simulink model "diffrelay"  (Simulink 8.5)
settings: Solver=ode45  SolverMode=SingleTasking  StartTime=0.0  StopTime=1.0  RelTol=1e-3  AbsTol=1e-6
undefined symbols (not defined in the file or in its folder): Time
libraries: elements x51
settings Model: Creator=PC  LastModifiedBy=PC  ExtModeTrigMode=oneshot  ExtModeArmWhenConnect=off
settings DataIOCC: LimitDataPoints=off
settings OptimizationCC: BlockReduction=off  BooleanDataType=off  ExpressionDepthLimit=128
settings DebuggingCC: SaveWithParameterizedLinksMsg=none  SignalResolutionControl=TryResolveAllWithWarning  MultiTaskDSMMsg=warning  MultiTaskCondExecSysMsg=none  FcnCallInpInsideContextMsg=EnableAllAsError  StateNameClashWarn=none
settings HardwareCC: TargetUnknown=on

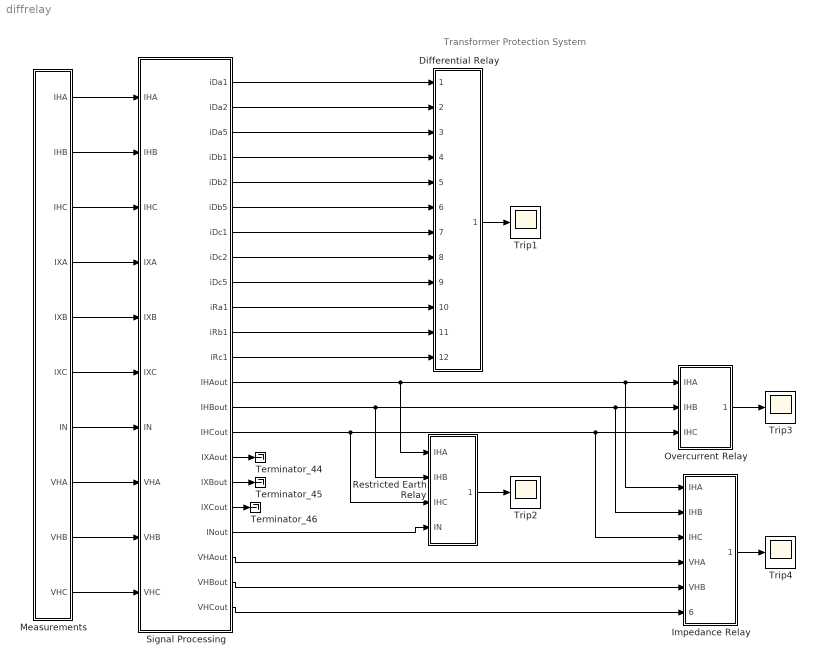
== system diffrelay ==
  note: Transformer Protection System
  Differential Relay : Subsystem  mask(Differential Relay){y2=300, x2=1000, y1=100, x1=500, c5=0.15, c2=0.15, unbiased=1e6, pickup=1}
      mask prompts: y2 "Biased Characteristic Point: D2"; x2 "Biased Characteristic Point: R2"; y1 "Biased Characteristic Point: D1"; x1 "Biased Characteristic Point: R1"; c5 "Fifth Harmonics Restraint Parameter"; c2 "Second Harmonics Restraint Parameter"; unbiased "Unbiased Threshold Value"; pickup "Pickup Value"
      mask help: Two-slope bias characteristic, instantaneous unbiased differential overcurrent element, second and fifth harmonic restraints.
  Impedance Relay : Subsystem  mask(Six-element Three-zone Impedance Relay){r=[0 0; -60 0; -65 -65; 0 -60], z2=[0 -0.5 ;1 0; 2 40; -0.5 0], z1=[0 -0.5 ;0.6 0; 1 21; -0.5 0]}
      mask prompts: r "Backward Zone Setting"; z2 "Zone 2 Setting"; z1 "Zone 1 Setting"
      mask help: Six-element three-zone (two forward and one backward) impedance relays for the backup protection of the high voltage winding.
  Measurements : Subsystem
  Overcurrent Relay : Subsystem  mask(Three-phase Inverse-time Overcurrent Relay){k=0.02, reset=0.9, pickupv=500}
      mask prompts: k "Time Parameter"; reset "Ratio of Reset to pick up"; pickupv "Pick-up Value"
      mask help: Three-phase inverse-time overcurrent relays for the back-up protection of the high voltage winding.
  Restricted Earth Relay : Subsystem  mask(Restricted Earth Protection for the Wye-connected Winding){rc=1, pickup0=0.5, zot=2100, k=0.2, choice=Differential}
      mask prompts: rc "Ratio Mismatch Compensation"; pickup0 "Zero Differential Pick-up Value"; zot "Zero Sequence Overcurrent Threshold"; k "Biased Parameter"; choice "Type of protection"
      mask help: Zero sequence overcurrent protection and zero sequence differential protection.
      mask TypeOptions choice: Overcurrent | Differential
  Signal Processing : Subsystem  mask(Signal Processing){ctx=31.5, cth=1.38, vs=13.8e3, vp=315e3, vector=11}
      mask prompts: ctx "CT Ratio of Low Voltage Side"; cth "CT Ratio of High Voltage Side"; vs "Secondary Voltage"; vp "Primary Voltage"; vector "Transformer Connection Vector"
      mask help: Transform analog measurements to digital format, including filtering, sampling . . .
  Terminator_44 : Terminator
  Terminator_45 : Terminator
  Terminator_46 : Terminator
  Trip{1..4} (4 alike) : Scope
      Trip1 settings: YMin=-1  YMax=1
      Trip2 settings: YMin=-2  YMax=2
      Trip3 settings: YMin=-1  YMax=1
      Trip4 settings: YMin=-1  YMax=1
  wires:
  Measurements/1(IHA) -> Signal Processing/1(IHA)
  Signal Processing/1(iDa1) -> Differential Relay/1(IDa1)
  Signal Processing/2(iDa2) -> Differential Relay/2(IDa2)
  Signal Processing/7(iDc1) -> Differential Relay/7(IDc1)
  Signal Processing/8(iDc2) -> Differential Relay/8(IDc2)
  Signal Processing/12(iRc1) -> Differential Relay/12(IRc1)
  Signal Processing/11(iRb1) -> Differential Relay/11(IRb1)
  Signal Processing/10(iRa1) -> Differential Relay/10(IRa1)
  Signal Processing/9(iDc5) -> Differential Relay/9(IDc5)
  Signal Processing/16(IXAout) -> Terminator_44/1
  Signal Processing/17(IXBout) -> Terminator_45/1
  Signal Processing/18(IXCout) -> Terminator_46/1
  Signal Processing/19(INout) -> Restricted Earth Relay/4(IN)
  Signal Processing/13(IHAout) -> Restricted Earth Relay/1(IHA), Overcurrent Relay/1(IHA), Impedance Relay/1(IHA)
  Signal Processing/14(IHBout) -> Restricted Earth Relay/2(IHB), Overcurrent Relay/2(IHB), Impedance Relay/2(IHB)
  Signal Processing/15(IHCout) -> Restricted Earth Relay/3(IHC), Overcurrent Relay/3(IHC), Impedance Relay/3(IHC)
  Signal Processing/20(VHAout) -> Impedance Relay/4(VHA)
  Signal Processing/21(VHBout) -> Impedance Relay/5(VHB)
  Signal Processing/22(VHCout) -> Impedance Relay/6(VHC)
  Measurements/2(IHB) -> Signal Processing/2(IHB)
  Measurements/3(IHC) -> Signal Processing/3(IHC)
  Measurements/4(IXA) -> Signal Processing/4(IXA)
  Measurements/5(IXB) -> Signal Processing/5(IXB)
  Measurements/6(IXC) -> Signal Processing/6(IXC)
  Measurements/7(IN) -> Signal Processing/7(IN)
  Measurements/8(VHA) -> Signal Processing/8(VHA)
  Measurements/9(VHB) -> Signal Processing/9(VHB)
  Measurements/10(VHC) -> Signal Processing/10(VHC)
  Differential Relay/1(Trip1) -> Trip1/1
  Overcurrent Relay/1(Trip 3) -> Trip3/1
  Restricted Earth Relay/1(Trip 2) -> Trip2/1
  Impedance Relay/1(Trip4) -> Trip4/1
  Signal Processing/3(iDa5) -> Differential Relay/3(IDa5)
  Signal Processing/4(iDb1) -> Differential Relay/4(IDb1)
  Signal Processing/5(iDb2) -> Differential Relay/5(IDb2)
  Signal Processing/6(iDb5) -> Differential Relay/6(IDb5)

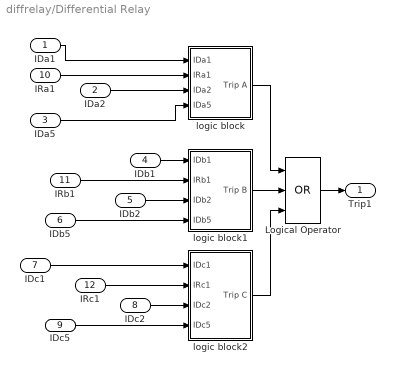
== system diffrelay/Differential Relay ==
  IDa1 : Inport
  IDa2 : Inport  Port=2
  IDa5 : Inport  Port=3
  IDb1 : Inport  Port=4
  IDb2 : Inport  Port=5
  IDb5 : Inport  Port=6
  IDc1 : Inport  Port=7
  IDc2 : Inport  Port=8
  IDc5 : Inport  Port=9
  IRa1 : Inport  Port=10
  IRb1 : Inport  Port=11
  IRc1 : Inport  Port=12
  Logical Operator : Logic  Operator=OR  Inputs=3
  logic block : Subsystem
  logic block1 : Subsystem
  logic block2 : Subsystem
  Trip1 : Outport
  wires:
  logic block/1(Trip A) -> Logical Operator/1
  logic block1/1(Trip B) -> Logical Operator/2
  logic block2/1(Trip C) -> Logical Operator/3
  Logical Operator/1 -> Trip1/1
  IRc1/1 -> logic block2/2(IRc1)
  IRb1/1 -> logic block1/2(IRb1)
  IDc5/1 -> logic block2/4(IDc5)
  IDc2/1 -> logic block2/3(IDc2)
  IDb2/1 -> logic block1/3(IDb2)
  IDb1/1 -> logic block1/1(IDb1)
  IDa5/1 -> logic block/4(IDa5)
  IDa2/1 -> logic block/3(IDa2)
  IDa1/1 -> logic block/1(IDa1)
  IRa1/1 -> logic block/2(IRa1)
  IDc1/1 -> logic block2/1(IDc1)
  IDb5/1 -> logic block1/4(IDb5)

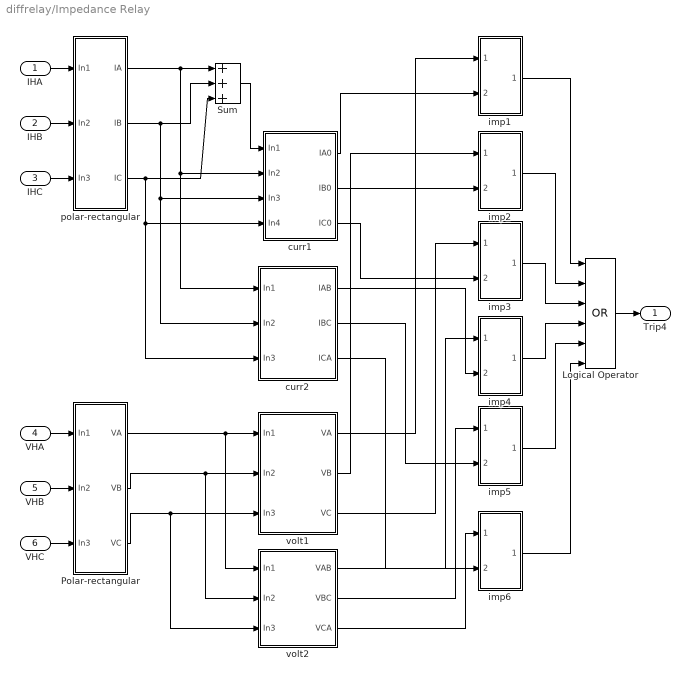
== system diffrelay/Impedance Relay ==
  IHA : Inport
  IHB : Inport  Port=2
  IHC : Inport  Port=3
  VHA : Inport  Port=4
  VHB : Inport  Port=5
  VHC : Inport  Port=6
  " curr1" : Subsystem
  Logical Operator : Logic  Operator=OR  Inputs=6
  Polar-rectangular : Subsystem
  Sum : Sum  Inputs=+++  SaturateOnIntegerOverflow=on  InputSameDT=on  OutDataTypeStr=Inherit: Same as first input
  curr2 : Subsystem
  imp1 : Subsystem
  imp2 : Subsystem
  imp3 : Subsystem
  imp4 : Subsystem
  imp5 : Subsystem
  imp6 : Subsystem
  polar-rectangular : Subsystem
  volt1 : Subsystem
  volt2 : Subsystem
  Trip4 : Outport
  wires:
  " curr1"/1(IA0) -> imp1/2(In2)
  polar-rectangular/1(IA) -> Sum/1, " curr1"/2(In2), curr2/1(In1)
  volt1/1(VA) -> imp1/1(In1)
  Polar-rectangular/1(VA) -> volt1/1(In1), volt2/1(In1)
  Polar-rectangular/2(VB) -> volt1/2(In2), volt2/2(In2)
  polar-rectangular/2(IB) -> Sum/2, " curr1"/3(In3), curr2/2(In2)
  polar-rectangular/3(IC) -> Sum/3, " curr1"/4(In4), curr2/3(In3)
  Polar-rectangular/3(VC) -> volt1/3(In3), volt2/3(In3)
  Sum/1 -> " curr1"/1(In1)
  imp1/1(e1trip) -> Logical Operator/1
  imp2/1(e2trip) -> Logical Operator/2
  imp3/1(e3trip) -> Logical Operator/3
  imp4/1(e4trip) -> Logical Operator/4
  imp5/1(e5trip) -> Logical Operator/5
  imp6/1(e6trip) -> Logical Operator/6
  Logical Operator/1 -> Trip4/1
  " curr1"/2(IB0) -> imp2/2(In2)
  volt1/2(VB) -> imp2/1(In1)
  volt1/3(VC) -> imp3/1(In1)
  " curr1"/3(IC0) -> imp3/2(In2)
  volt2/1(VAB) -> imp4/1(In1)
  curr2/1(IAB) -> imp4/2(In2)
  volt2/2(VBC) -> imp5/1(In1)
  curr2/2(IBC) -> imp5/2(In2)
  volt2/3(VCA) -> imp6/1(In1)
  curr2/3(ICA) -> imp6/2(In2)
  IHA/1 -> polar-rectangular/1(In1)
  IHB/1 -> polar-rectangular/2(In2)
  IHC/1 -> polar-rectangular/3(In3)
  VHA/1 -> Polar-rectangular/1(In1)
  VHB/1 -> Polar-rectangular/2(In2)
  VHC/1 -> Polar-rectangular/3(In3)

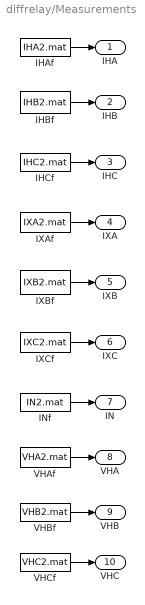
== system diffrelay/Measurements ==
  IHAf : FromFile  FileName=IHA2.mat  SampleTime=0
  IHBf : FromFile  FileName=IHB2.mat  SampleTime=0
  IHCf : FromFile  FileName=IHC2.mat  SampleTime=0
  INf : FromFile  FileName=IN2.mat  SampleTime=0
  IXAf : FromFile  FileName=IXA2.mat  SampleTime=0
  IXBf : FromFile  FileName=IXB2.mat  SampleTime=0
  IXCf : FromFile  FileName=IXC2.mat  SampleTime=0
  VHAf : FromFile  FileName=VHA2.mat  SampleTime=0
  VHBf : FromFile  FileName=VHB2.mat  SampleTime=0
  VHCf : FromFile  FileName=VHC2.mat  SampleTime=0
  IHA : Outport
  IHB : Outport  Port=2
  IHC : Outport  Port=3
  IXA : Outport  Port=4
  IXB : Outport  Port=5
  IXC : Outport  Port=6
  IN : Outport  Port=7
  VHA : Outport  Port=8
  VHB : Outport  Port=9
  VHC : Outport  Port=10
  wires:
  IHAf/1 -> IHA/1
  IHBf/1 -> IHB/1
  IHCf/1 -> IHC/1
  IXAf/1 -> IXA/1
  IXBf/1 -> IXB/1
  IXCf/1 -> IXC/1
  INf/1 -> IN/1
  VHAf/1 -> VHA/1
  VHBf/1 -> VHB/1
  VHCf/1 -> VHC/1

== system diffrelay/Overcurrent Relay ==
  IHA : Inport
  IHB : Inport  Port=2
  IHC : Inport  Port=3
  Demux : Demux  Outputs=2
  Demux1 : Demux  Outputs=2
  Demux2 : Demux  Outputs=2
  Logical Operator : Logic  Operator=OR  Inputs=3
  UCA : elements/UC  type0=Signal-Time  sign=>  Ipickup=pickupv  k1=reset  type1=Very Inverse  type3=integration  k=k  fs=32*60
  UCB : elements/UC  type0=Signal-Time  sign=>  Ipickup=pickupv  k1=reset  type1=Very Inverse  type3=integration  k=k  fs=32*60
  UCC : elements/UC  type0=Signal-Time  sign=>  Ipickup=pickupv  k1=reset  type1=Very Inverse  type3=integration  k=k  fs=32*60
  Trip 3 : Outport
  wires:
  Demux2/1 -> UCC/1
  Demux1/1 -> UCB/1
  Demux/1 -> UCA/1
  UCA/1 -> Logical Operator/1
  UCB/1 -> Logical Operator/2
  UCC/1 -> Logical Operator/3
  Logical Operator/1 -> Trip 3/1
  IHA/1 -> Demux/1
  IHB/1 -> Demux1/1
  IHC/1 -> Demux2/1
  Demux/2 -> UCA/2
  Demux1/2 -> UCB/2
  Demux2/2 -> UCC/2

== system diffrelay/Restricted Earth Relay ==
  IHA : Inport
  IHB : Inport  Port=2
  IHC : Inport  Port=3
  IN : Inport  Port=4
  Choice : Constant  Value=choice
  Switch : Switch  Threshold=1.5  SaturateOnIntegerOverflow=on  InputSameDT=on
  Zero Sequence Differential : Subsystem
  Zero Sequence  Overcurrent : Subsystem
  rc : Gain  Gain=rc  SaturateOnIntegerOverflow=on  OutDataTypeStr=Inherit: Same as input  ParamDataTypeStr=Inherit: Same as input
  Trip 2 : Outport
  wires:
  Choice/1 -> Switch/2
  Zero Sequence Differential/1(Out1) -> Switch/1
  Switch/1 -> Trip 2/1
  Zero Sequence  Overcurrent/1(Out1) -> Switch/3
  IHA/1 -> Zero Sequence Differential/1(IHA)
  IHB/1 -> Zero Sequence Differential/2(IHB)
  IHC/1 -> Zero Sequence Differential/3(IHC)
  IN/1 -> Zero Sequence  Overcurrent/1(In1), rc/1
  rc/1 -> Zero Sequence Differential/4(IN)

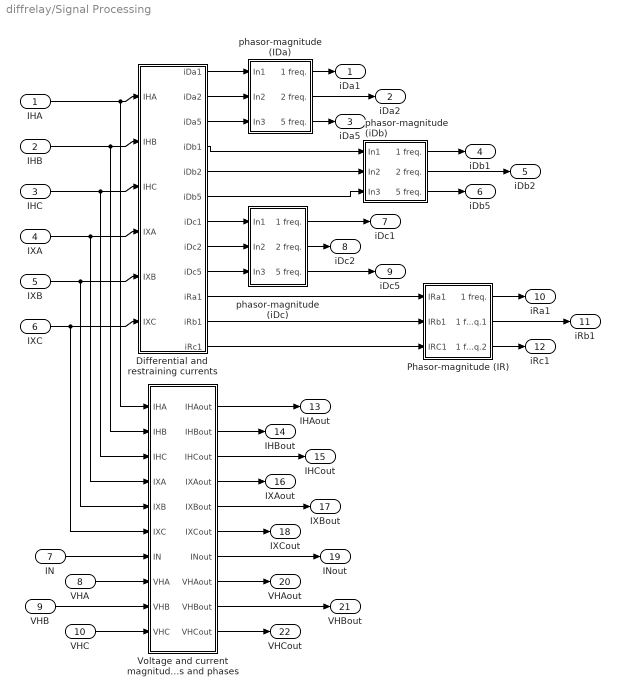
== system diffrelay/Signal Processing ==
  IHA : Inport
  IHB : Inport  Port=2
  IHC : Inport  Port=3
  IXA : Inport  Port=4
  IXB : Inport  Port=5
  IXC : Inport  Port=6
  IN : Inport  Port=7
  VHA : Inport  Port=8
  VHB : Inport  Port=9
  VHC : Inport  Port=10
  Differential and  restraining currents : Subsystem
  Phasor-magnitude (IR) : Subsystem
  Voltage and current magnitudes and phases : Subsystem
  phasor-magnitude (IDa) : Subsystem
  phasor-magnitude (iDb) : Subsystem
  phasor-magnitude (iDc) : Subsystem
  iDa1 : Outport
  iDa2 : Outport  Port=2
  iDa5 : Outport  Port=3
  iDb1 : Outport  Port=4
  iDb2 : Outport  Port=5
  iDb5 : Outport  Port=6
  iDc1 : Outport  Port=7
  iDc2 : Outport  Port=8
  iDc5 : Outport  Port=9
  iRa1 : Outport  Port=10
  iRb1 : Outport  Port=11
  iRc1 : Outport  Port=12
  IHAout : Outport  Port=13
  IHBout : Outport  Port=14
  IHCout : Outport  Port=15
  IXAout : Outport  Port=16
  IXBout : Outport  Port=17
  IXCout : Outport  Port=18
  INout : Outport  Port=19
  VHAout : Outport  Port=20
  VHBout : Outport  Port=21
  VHCout : Outport  Port=22
  wires:
  IHA/1 -> Differential and  restraining currents/1(IHA), Voltage and current magnitudes and phases/1(IHA)
  IHB/1 -> Differential and  restraining currents/2(IHB), Voltage and current magnitudes and phases/2(IHB)
  IHC/1 -> Differential and  restraining currents/3(IHC), Voltage and current magnitudes and phases/3(IHC)
  IXA/1 -> Differential and  restraining currents/4(IXA), Voltage and current magnitudes and phases/4(IXA)
  IXB/1 -> Differential and  restraining currents/5(IXB), Voltage and current magnitudes and phases/5(IXB)
  IXC/1 -> Differential and  restraining currents/6(IXC), Voltage and current magnitudes and phases/6(IXC)
  Differential and  restraining currents/1(iDa1) -> phasor-magnitude (IDa)/1(In1)
  Differential and  restraining currents/2(iDa2) -> phasor-magnitude (IDa)/2(In2)
  Differential and  restraining currents/3(iDa5) -> phasor-magnitude (IDa)/3(In3)
  phasor-magnitude (IDa)/1(1 freq.) -> iDa1/1
  phasor-magnitude (IDa)/2(2 freq.) -> iDa2/1
  phasor-magnitude (IDa)/3(5 freq.) -> iDa5/1
  Differential and  restraining currents/4(iDb1) -> phasor-magnitude (iDb)/1(In1)
  Differential and  restraining currents/5(iDb2) -> phasor-magnitude (iDb)/2(In2)
  Differential and  restraining currents/6(iDb5) -> phasor-magnitude (iDb)/3(In3)
  phasor-magnitude (iDb)/1(1 freq.) -> iDb1/1
  phasor-magnitude (iDb)/2(2 freq.) -> iDb2/1
  phasor-magnitude (iDb)/3(5 freq.) -> iDb5/1
  Differential and  restraining currents/7(iDc1) -> phasor-magnitude (iDc)/1(In1)
  Differential and  restraining currents/8(iDc2) -> phasor-magnitude (iDc)/2(In2)
  Differential and  restraining currents/9(iDc5) -> phasor-magnitude (iDc)/3(In3)
  phasor-magnitude (iDc)/1(1 freq.) -> iDc1/1
  phasor-magnitude (iDc)/2(2 freq.) -> iDc2/1
  phasor-magnitude (iDc)/3(5 freq.) -> iDc5/1
  Differential and  restraining currents/10(iRa1) -> Phasor-magnitude (IR)/1(IRa1)
  Differential and  restraining currents/11(iRb1) -> Phasor-magnitude (IR)/2(IRb1)
  Differential and  restraining currents/12(iRc1) -> Phasor-magnitude (IR)/3(IRC1)
  Phasor-magnitude (IR)/1(1 freq.) -> iRa1/1
  Phasor-magnitude (IR)/2(1 freq.1) -> iRb1/1
  Phasor-magnitude (IR)/3(1 freq.2) -> iRc1/1
  Voltage and current magnitudes and phases/1(IHAout) -> IHAout/1
  Voltage and current magnitudes and phases/2(IHBout) -> IHBout/1
  Voltage and current magnitudes and phases/3(IHCout) -> IHCout/1
  Voltage and current magnitudes and phases/4(IXAout) -> IXAout/1
  Voltage and current magnitudes and phases/5(IXBout) -> IXBout/1
  Voltage and current magnitudes and phases/6(IXCout) -> IXCout/1
  Voltage and current magnitudes and phases/7(INout) -> INout/1
  Voltage and current magnitudes and phases/8(VHAout) -> VHAout/1
  Voltage and current magnitudes and phases/9(VHBout) -> VHBout/1
  Voltage and current magnitudes and phases/10(VHCout) -> VHCout/1
  IN/1 -> Voltage and current magnitudes and phases/7(IN)
  VHA/1 -> Voltage and current magnitudes and phases/8(VHA)
  VHB/1 -> Voltage and current magnitudes and phases/9(VHB)
  VHC/1 -> Voltage and current magnitudes and phases/10(VHC)

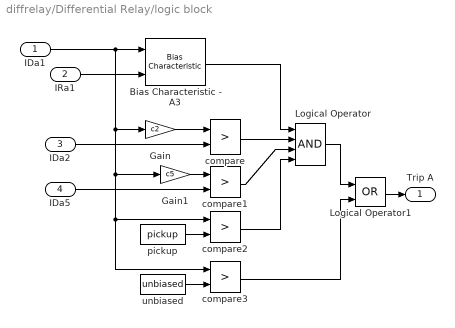
== system diffrelay/Differential Relay/logic block ==
  IDa1 : Inport
  IRa1 : Inport  Port=2
  IDa2 : Inport  Port=3
  IDa5 : Inport  Port=4
  Bias Characteristic - A3 : elements/Bias Characteristic  BC=[ 0 0; x1 y1; x2 y2 ]  fs=60*32
  Gain : Gain  Gain=c2  SaturateOnIntegerOverflow=on  OutDataTypeStr=Inherit: Same as input  ParamDataTypeStr=Inherit: Same as input
  Gain1 : Gain  Gain=c5  SaturateOnIntegerOverflow=on  OutDataTypeStr=Inherit: Same as input  ParamDataTypeStr=Inherit: Same as input
  Logical Operator : Logic  Inputs=4
  Logical Operator1 : Logic  Operator=OR
  compare{,1..3} (4 alike) : RelationalOperator  Operator=>  InputSameDT=on
  pickup : Constant  Value=pickup
  unbiased : Constant  Value=unbiased
  Trip A : Outport
  wires:
  Gain/1 -> compare/1
  Gain1/1 -> compare1/1
  pickup/1 -> compare2/2
  unbiased/1 -> compare3/2
  IDa2/1 -> compare/2
  IDa5/1 -> compare1/2
  Logical Operator1/1 -> Trip A/1
  Logical Operator/1 -> Logical Operator1/1
  compare3/1 -> Logical Operator1/2
  Bias Characteristic - A3/1 -> Logical Operator/1
  compare/1 -> Logical Operator/2
  compare1/1 -> Logical Operator/3
  compare2/1 -> Logical Operator/4
  IRa1/1 -> Bias Characteristic - A3/2
  IDa1/1 -> Bias Characteristic - A3/1, Gain/1, Gain1/1, compare2/1, compare3/1

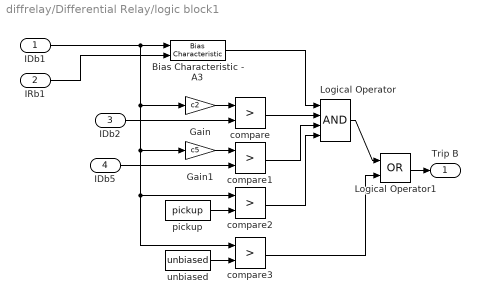
== system diffrelay/Differential Relay/logic block1 ==
  IDb1 : Inport
  IRb1 : Inport  Port=2
  IDb2 : Inport  Port=3
  IDb5 : Inport  Port=4
  Bias Characteristic - A3 : elements/Bias Characteristic  BC=[ 0 0; x1 y1; x2 y2 ]  fs=60*32
  Gain : Gain  Gain=c2  SaturateOnIntegerOverflow=on  OutDataTypeStr=Inherit: Same as input  ParamDataTypeStr=Inherit: Same as input
  Gain1 : Gain  Gain=c5  SaturateOnIntegerOverflow=on  OutDataTypeStr=Inherit: Same as input  ParamDataTypeStr=Inherit: Same as input
  Logical Operator : Logic  Inputs=4
  Logical Operator1 : Logic  Operator=OR
  compare{,1..3} (4 alike) : RelationalOperator  Operator=>  InputSameDT=on
  pickup : Constant  Value=pickup
  unbiased : Constant  Value=unbiased
  Trip B : Outport
  wires:
  IDb1/1 -> compare3/1, compare2/1, Gain1/1, Gain/1, Bias Characteristic - A3/1
  IRb1/1 -> Bias Characteristic - A3/2
  compare2/1 -> Logical Operator/4
  compare1/1 -> Logical Operator/3
  compare/1 -> Logical Operator/2
  Bias Characteristic - A3/1 -> Logical Operator/1
  compare3/1 -> Logical Operator1/2
  Logical Operator/1 -> Logical Operator1/1
  Logical Operator1/1 -> Trip B/1
  IDb5/1 -> compare1/2
  IDb2/1 -> compare/2
  unbiased/1 -> compare3/2
  pickup/1 -> compare2/2
  Gain1/1 -> compare1/1
  Gain/1 -> compare/1

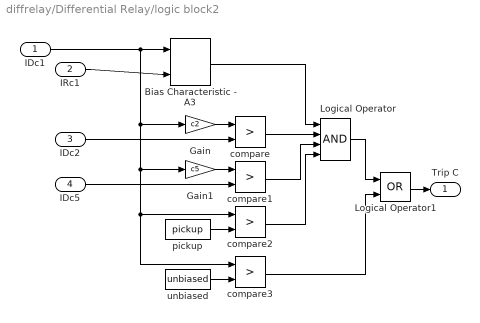
== system diffrelay/Differential Relay/logic block2 ==
  IDc1 : Inport
  IRc1 : Inport  Port=2
  IDc2 : Inport  Port=3
  IDc5 : Inport  Port=4
  Bias Characteristic - A3 : elements/Bias Characteristic  BC=[ 0 0; x1 y1; x2 y2 ]  fs=60*32
  Gain : Gain  Gain=c2  SaturateOnIntegerOverflow=on  OutDataTypeStr=Inherit: Same as input  ParamDataTypeStr=Inherit: Same as input
  Gain1 : Gain  Gain=c5  SaturateOnIntegerOverflow=on  OutDataTypeStr=Inherit: Same as input  ParamDataTypeStr=Inherit: Same as input
  Logical Operator : Logic  Inputs=4
  Logical Operator1 : Logic  Operator=OR
  compare{,1..3} (4 alike) : RelationalOperator  Operator=>  InputSameDT=on
  pickup : Constant  Value=pickup
  unbiased : Constant  Value=unbiased
  Trip C : Outport
  wires:
  Gain/1 -> compare/1
  Gain1/1 -> compare1/1
  pickup/1 -> compare2/2
  unbiased/1 -> compare3/2
  IDc2/1 -> compare/2
  IDc5/1 -> compare1/2
  Logical Operator1/1 -> Trip C/1
  Logical Operator/1 -> Logical Operator1/1
  compare3/1 -> Logical Operator1/2
  Bias Characteristic - A3/1 -> Logical Operator/1
  compare/1 -> Logical Operator/2
  compare1/1 -> Logical Operator/3
  compare2/1 -> Logical Operator/4
  IRc1/1 -> Bias Characteristic - A3/2
  IDc1/1 -> Bias Characteristic - A3/1, Gain/1, Gain1/1, compare2/1, compare3/1

== system diffrelay/Impedance Relay/ curr1 ==
  In1 : Inport
  In2 : Inport  Port=2
  In3 : Inport  Port=3
  In4 : Inport  Port=4
  C to M/A : Subsystem
  C to M/A1 : Subsystem
  C to M/A2 : Subsystem
  Sum1 : Sum  Inputs=2  SaturateOnIntegerOverflow=on  InputSameDT=on  OutDataTypeStr=Inherit: Same as first input
  Sum2 : Sum  Inputs=2  SaturateOnIntegerOverflow=on  InputSameDT=on  OutDataTypeStr=Inherit: Same as first input
  Sum3 : Sum  Inputs=2  SaturateOnIntegerOverflow=on  InputSameDT=on  OutDataTypeStr=Inherit: Same as first input
  IA0 : Outport
  IB0 : Outport  Port=2
  IC0 : Outport  Port=3
  wires:
  In1/1 -> Sum1/1, Sum2/1, Sum3/1
  Sum1/1 -> C to M/A/1(In1)
  In3/1 -> Sum2/2
  In2/1 -> Sum1/2
  Sum2/1 -> C to M/A1/1(In1)
  Sum3/1 -> C to M/A2/1(In1)
  In4/1 -> Sum3/2
  C to M/A/1(Out1) -> IA0/1
  C to M/A1/1(Out1) -> IB0/1
  C to M/A2/1(Out1) -> IC0/1

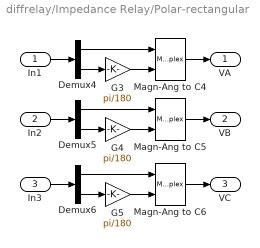
== system diffrelay/Impedance Relay/Polar-rectangular ==
  In1 : Inport
  In2 : Inport  Port=2
  In3 : Inport  Port=3
  Demux4 : Demux  Outputs=2
  Demux5 : Demux  Outputs=2
  Demux6 : Demux  Outputs=2
  G3 : Gain  Gain=pi/180  SaturateOnIntegerOverflow=on  OutDataTypeStr=Inherit: Same as input  ParamDataTypeStr=Inherit: Same as input
  G4 : Gain  Gain=pi/180  SaturateOnIntegerOverflow=on  OutDataTypeStr=Inherit: Same as input  ParamDataTypeStr=Inherit: Same as input
  G5 : Gain  Gain=pi/180  SaturateOnIntegerOverflow=on  OutDataTypeStr=Inherit: Same as input  ParamDataTypeStr=Inherit: Same as input
  Magn-Ang to C4 : MagnitudeAngleToComplex
  Magn-Ang to C5 : MagnitudeAngleToComplex
  Magn-Ang to C6 : MagnitudeAngleToComplex
  VA : Outport
  VB : Outport  Port=2
  VC : Outport  Port=3
  wires:
  Demux4/1 -> Magn-Ang to C4/1
  Demux4/2 -> G3/1
  G3/1 -> Magn-Ang to C4/2
  Demux5/2 -> G4/1
  G4/1 -> Magn-Ang to C5/2
  Demux5/1 -> Magn-Ang to C5/1
  Demux6/2 -> G5/1
  G5/1 -> Magn-Ang to C6/2
  Demux6/1 -> Magn-Ang to C6/1
  Magn-Ang to C4/1 -> VA/1
  In1/1 -> Demux4/1
  Magn-Ang to C5/1 -> VB/1
  In2/1 -> Demux5/1
  Magn-Ang to C6/1 -> VC/1
  In3/1 -> Demux6/1

== system diffrelay/Impedance Relay/curr2 ==
  In1 : Inport
  In2 : Inport  Port=2
  In3 : Inport  Port=3
  C to M/A : Subsystem
  C to M/A1 : Subsystem
  C to M/A2 : Subsystem
  Sum4 : Sum  Inputs=+-  SaturateOnIntegerOverflow=on  InputSameDT=on  OutDataTypeStr=Inherit: Same as first input
  Sum6 : Sum  Inputs=+-  SaturateOnIntegerOverflow=on  InputSameDT=on  OutDataTypeStr=Inherit: Same as first input
  Sum7 : Sum  Inputs=+-  SaturateOnIntegerOverflow=on  InputSameDT=on  OutDataTypeStr=Inherit: Same as first input
  IAB : Outport
  IBC : Outport  Port=2
  ICA : Outport  Port=3
  wires:
  In2/1 -> Sum4/2, Sum6/1
  In3/1 -> Sum6/2, Sum7/1
  In1/1 -> Sum4/1, Sum7/2
  Sum4/1 -> C to M/A/1(In1)
  C to M/A/1(Out1) -> IAB/1
  Sum6/1 -> C to M/A1/1(In1)
  C to M/A1/1(Out1) -> IBC/1
  Sum7/1 -> C to M/A2/1(In1)
  C to M/A2/1(Out1) -> ICA/1

== system diffrelay/Impedance Relay/imp1 ==
  In1 : Inport
  In2 : Inport  Port=2
   {,1,3..5} (5 alike) : Terminator
  BM : elements/BM  tpostv=none  plenv=4  tposti=none  pleni=4  tposts=none  plens=4  tpostz=none  plenz=4
  Logical Operator : Logic  Operator=OR  Inputs=3
  Time Delay1 : TransportDelay  DelayTime=0.2  BufferSize=2048
  Time Delay2 : TransportDelay  DelayTime=0.5  BufferSize=4096
  "ZC   " : elements/ZC     typez=Free expression  z1=z1  z2=z2  z3="[0  0; 0 0; 0 0; 0 0]"  z4="[0  0; 0 0; 0 0; 0 0]"  zr=r  fs=32*60
  e1trip : Outport
  wires:
  "ZC   "/2 -> Time Delay1/1
  "ZC   "/5 -> Time Delay2/1
  "ZC   "/3 -> " 3"/1
  "ZC   "/4 -> " 4"/1
  Time Delay1/1 -> Logical Operator/2
  Time Delay2/1 -> Logical Operator/3
  Logical Operator/1 -> e1trip/1
  BM/1 -> " "/1
  BM/2 -> " 1"/1
  BM/3 -> " 5"/1
  In1/1 -> BM/1
  In2/1 -> BM/2
  BM/4 -> "ZC   "/1
  "ZC   "/1 -> Logical Operator/1

== system diffrelay/Impedance Relay/imp2 ==
  In1 : Inport
  In2 : Inport  Port=2
   {,1,3..5} (5 alike) : Terminator
  BM : elements/BM  tpostv=none  plenv=4  tposti=none  pleni=4  tposts=none  plens=4  tpostz=none  plenz=4
  Logical Operator : Logic  Operator=OR  Inputs=3
  Time Delay1 : TransportDelay  DelayTime=0.2  BufferSize=2048
  Time Delay2 : TransportDelay  DelayTime=0.5  BufferSize=4096
  "ZC   " : elements/ZC     typez=Free expression  z1=z1  z2=z2  z3="[0  0; 0 0; 0 0; 0 0]"  z4="[0  0; 0 0; 0 0; 0 0]"  zr=r  fs=32*60
  e2trip : Outport
  wires:
  "ZC   "/1 -> Logical Operator/1
  BM/4 -> "ZC   "/1
  In2/1 -> BM/2
  In1/1 -> BM/1
  BM/3 -> " 5"/1
  BM/2 -> " 1"/1
  BM/1 -> " "/1
  Logical Operator/1 -> e2trip/1
  Time Delay2/1 -> Logical Operator/3
  Time Delay1/1 -> Logical Operator/2
  "ZC   "/4 -> " 4"/1
  "ZC   "/3 -> " 3"/1
  "ZC   "/5 -> Time Delay2/1
  "ZC   "/2 -> Time Delay1/1

== system diffrelay/Impedance Relay/imp3 ==
  In1 : Inport
  In2 : Inport  Port=2
   {,1,3..5} (5 alike) : Terminator
  BM : elements/BM  tpostv=none  plenv=4  tposti=none  pleni=4  tposts=none  plens=4  tpostz=none  plenz=4
  Logical Operator : Logic  Operator=OR  Inputs=3
  Time Delay1 : TransportDelay  DelayTime=0.2  BufferSize=2048
  Time Delay2 : TransportDelay  DelayTime=0.5  BufferSize=4096
  "ZC   " : elements/ZC     typez=Free expression  z1=z1  z2=z2  z3="[0  0; 0 0; 0 0; 0 0]"  z4="[0  0; 0 0; 0 0; 0 0]"  zr=r  fs=32*60
  e3trip : Outport
  wires:
  "ZC   "/2 -> Time Delay1/1
  "ZC   "/5 -> Time Delay2/1
  "ZC   "/3 -> " 3"/1
  "ZC   "/4 -> " 4"/1
  Time Delay1/1 -> Logical Operator/2
  Time Delay2/1 -> Logical Operator/3
  Logical Operator/1 -> e3trip/1
  BM/1 -> " "/1
  BM/2 -> " 1"/1
  BM/3 -> " 5"/1
  In1/1 -> BM/1
  In2/1 -> BM/2
  BM/4 -> "ZC   "/1
  "ZC   "/1 -> Logical Operator/1

== system diffrelay/Impedance Relay/imp4 ==
  In1 : Inport
  In2 : Inport  Port=2
   {,1,3..5} (5 alike) : Terminator
  BM : elements/BM  tpostv=none  plenv=4  tposti=none  pleni=4  tposts=none  plens=4  tpostz=none  plenz=4
  Logical Operator : Logic  Operator=OR  Inputs=3
  Time Delay1 : TransportDelay  DelayTime=0.2  BufferSize=2048
  Time Delay2 : TransportDelay  DelayTime=0.5  BufferSize=4096
  "ZC   " : elements/ZC     typez=Free expression  z1=z1  z2=z2  z3="[0  0; 0 0; 0 0; 0 0]"  z4="[0  0; 0 0; 0 0; 0 0]"  zr=r  fs=32*60
  e4trip : Outport
  wires:
  "ZC   "/1 -> Logical Operator/1
  BM/4 -> "ZC   "/1
  In2/1 -> BM/2
  In1/1 -> BM/1
  BM/3 -> " 5"/1
  BM/2 -> " 1"/1
  BM/1 -> " "/1
  Logical Operator/1 -> e4trip/1
  Time Delay2/1 -> Logical Operator/3
  Time Delay1/1 -> Logical Operator/2
  "ZC   "/4 -> " 4"/1
  "ZC   "/3 -> " 3"/1
  "ZC   "/5 -> Time Delay2/1
  "ZC   "/2 -> Time Delay1/1

== system diffrelay/Impedance Relay/imp5 ==
  In1 : Inport
  In2 : Inport  Port=2
   {,1,3..5} (5 alike) : Terminator
  BM : elements/BM  tpostv=none  plenv=4  tposti=none  pleni=4  tposts=none  plens=4  tpostz=none  plenz=4
  Logical Operator : Logic  Operator=OR  Inputs=3
  Time Delay1 : TransportDelay  DelayTime=0.2  BufferSize=2048
  Time Delay2 : TransportDelay  DelayTime=0.5  BufferSize=4096
  "ZC   " : elements/ZC     typez=Free expression  z1=z1  z2=z2  z3="[0  0; 0 0; 0 0; 0 0]"  z4="[0  0; 0 0; 0 0; 0 0]"  zr=r  fs=32*60
  e5trip : Outport
  wires:
  "ZC   "/2 -> Time Delay1/1
  "ZC   "/5 -> Time Delay2/1
  "ZC   "/3 -> " 3"/1
  "ZC   "/4 -> " 4"/1
  Time Delay1/1 -> Logical Operator/2
  Time Delay2/1 -> Logical Operator/3
  Logical Operator/1 -> e5trip/1
  BM/1 -> " "/1
  BM/2 -> " 1"/1
  BM/3 -> " 5"/1
  In1/1 -> BM/1
  In2/1 -> BM/2
  BM/4 -> "ZC   "/1
  "ZC   "/1 -> Logical Operator/1

== system diffrelay/Impedance Relay/imp6 ==
  In1 : Inport
  In2 : Inport  Port=2
   {,1,3..5} (5 alike) : Terminator
  BM : elements/BM  tpostv=none  plenv=4  tposti=none  pleni=4  tposts=none  plens=4  tpostz=none  plenz=4
  Logical Operator : Logic  Operator=OR  Inputs=3
  Time Delay1 : TransportDelay  DelayTime=0.2  BufferSize=2048
  Time Delay2 : TransportDelay  DelayTime=0.5  BufferSize=4096
  "ZC   " : elements/ZC     typez=Free expression  z1=z1  z2=z2  z3="[0  0; 0 0; 0 0; 0 0]"  z4="[0  0; 0 0; 0 0; 0 0]"  zr=r  fs=32*60
  e6trip : Outport
  wires:
  "ZC   "/1 -> Logical Operator/1
  BM/4 -> "ZC   "/1
  In2/1 -> BM/2
  In1/1 -> BM/1
  BM/3 -> " 5"/1
  BM/2 -> " 1"/1
  BM/1 -> " "/1
  Logical Operator/1 -> e6trip/1
  Time Delay2/1 -> Logical Operator/3
  Time Delay1/1 -> Logical Operator/2
  "ZC   "/4 -> " 4"/1
  "ZC   "/3 -> " 3"/1
  "ZC   "/5 -> Time Delay2/1
  "ZC   "/2 -> Time Delay1/1

== system diffrelay/Impedance Relay/polar-rectangular ==
  In1 : Inport
  In2 : Inport  Port=2
  In3 : Inport  Port=3
  Demux1 : Demux  Outputs=2
  Demux2 : Demux  Outputs=2
  Demux3 : Demux  Outputs=2
  G : Gain  Gain=pi/180  SaturateOnIntegerOverflow=on  OutDataTypeStr=Inherit: Same as input  ParamDataTypeStr=Inherit: Same as input
  G1 : Gain  Gain=pi/180  SaturateOnIntegerOverflow=on  OutDataTypeStr=Inherit: Same as input  ParamDataTypeStr=Inherit: Same as input
  G2 : Gain  Gain=pi/180  SaturateOnIntegerOverflow=on  OutDataTypeStr=Inherit: Same as input  ParamDataTypeStr=Inherit: Same as input
  Magn-Ang to C1 : MagnitudeAngleToComplex
  Magn-Ang to C2 : MagnitudeAngleToComplex
  Magn-Ang to C3 : MagnitudeAngleToComplex
  IA : Outport
  IB : Outport  Port=2
  IC : Outport  Port=3
  wires:
  Demux1/2 -> G/1
  G/1 -> Magn-Ang to C1/2
  Demux1/1 -> Magn-Ang to C1/1
  Demux2/2 -> G1/1
  G1/1 -> Magn-Ang to C2/2
  Demux2/1 -> Magn-Ang to C2/1
  Demux3/2 -> G2/1
  G2/1 -> Magn-Ang to C3/2
  Demux3/1 -> Magn-Ang to C3/1
  Magn-Ang to C1/1 -> IA/1
  In1/1 -> Demux1/1
  Magn-Ang to C2/1 -> IB/1
  In2/1 -> Demux2/1
  Magn-Ang to C3/1 -> IC/1
  In3/1 -> Demux3/1

== system diffrelay/Impedance Relay/volt1 ==
  In1 : Inport
  In2 : Inport  Port=2
  In3 : Inport  Port=3
  C to M/A3 : Subsystem
  C to M/A4 : Subsystem
  C to M/A5 : Subsystem
  VA : Outport
  VB : Outport  Port=2
  VC : Outport  Port=3
  wires:
  In1/1 -> C to M/A3/1(In1)
  In2/1 -> C to M/A4/1(In1)
  In3/1 -> C to M/A5/1(In1)
  C to M/A3/1(Out1) -> VA/1
  C to M/A4/1(Out1) -> VB/1
  C to M/A5/1(Out1) -> VC/1

== system diffrelay/Impedance Relay/volt2 ==
  In1 : Inport
  In2 : Inport  Port=2
  In3 : Inport  Port=3
  C to M/A6 : Subsystem
  C to M/A7 : Subsystem
  C to M/A8 : Subsystem
  Sum5 : Sum  Inputs=+-  SaturateOnIntegerOverflow=on  InputSameDT=on  OutDataTypeStr=Inherit: Same as first input
  Sum8 : Sum  Inputs=+-  SaturateOnIntegerOverflow=on  InputSameDT=on  OutDataTypeStr=Inherit: Same as first input
  Sum9 : Sum  Inputs=+-  SaturateOnIntegerOverflow=on  InputSameDT=on  OutDataTypeStr=Inherit: Same as first input
  VAB : Outport
  VBC : Outport  Port=2
  VCA : Outport  Port=3
  wires:
  In2/1 -> Sum5/2, Sum8/1
  In3/1 -> Sum8/2, Sum9/1
  In1/1 -> Sum5/1, Sum9/2
  Sum5/1 -> C to M/A6/1(In1)
  Sum8/1 -> C to M/A7/1(In1)
  Sum9/1 -> C to M/A8/1(In1)
  C to M/A6/1(Out1) -> VAB/1
  C to M/A7/1(Out1) -> VBC/1
  C to M/A8/1(Out1) -> VCA/1

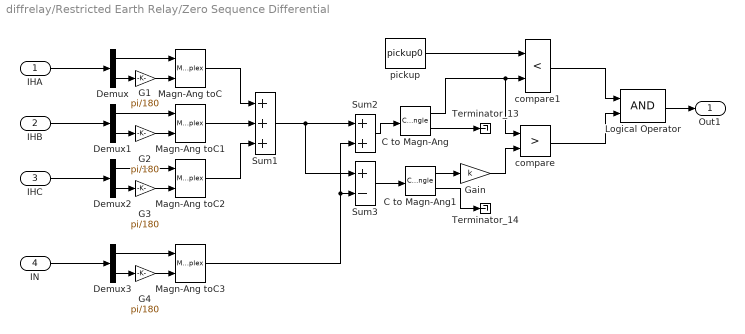
== system diffrelay/Restricted Earth Relay/Zero Sequence Differential ==
  IHA : Inport
  IHB : Inport  Port=2
  IHC : Inport  Port=3
  IN : Inport  Port=4
  C to Magn-Ang : ComplexToMagnitudeAngle
  C to Magn-Ang1 : ComplexToMagnitudeAngle
  Demux{,1..3} (4 alike) : Demux  Outputs=2
  G{1..4} (4 alike) : Gain  Gain=pi/180  SaturateOnIntegerOverflow=on  OutDataTypeStr=Inherit: Same as input  ParamDataTypeStr=Inherit: Same as input
  Gain : Gain  Gain=k  SaturateOnIntegerOverflow=on  OutDataTypeStr=Inherit: Same as input  ParamDataTypeStr=Inherit: Same as input
  Logical Operator : Logic
  Magn-Ang toC{,1..3} (4 alike) : MagnitudeAngleToComplex
  Sum1 : Sum  Inputs=+++  SaturateOnIntegerOverflow=on  InputSameDT=on  OutDataTypeStr=Inherit: Same as first input
  Sum2 : Sum  SaturateOnIntegerOverflow=on  InputSameDT=on  OutDataTypeStr=Inherit: Same as first input
  Sum3 : Sum  Inputs=+-  SaturateOnIntegerOverflow=on  InputSameDT=on  OutDataTypeStr=Inherit: Same as first input
  Terminator_13 : Terminator
  Terminator_14 : Terminator
  compare : RelationalOperator  Operator=>  InputSameDT=on
  compare1 : RelationalOperator  Operator=<  InputSameDT=on
  pickup : Constant  Value=pickup0
  Out1 : Outport
  wires:
  Sum2/1 -> C to Magn-Ang/1
  Sum3/1 -> C to Magn-Ang1/1
  IN/1 -> Demux3/1
  Demux3/1 -> Magn-Ang toC3/1
  Magn-Ang toC3/1 -> Sum3/2, Sum2/2
  C to Magn-Ang/2 -> Terminator_13/1
  C to Magn-Ang1/2 -> Terminator_14/1
  C to Magn-Ang1/1 -> Gain/1
  Gain/1 -> compare/2
  Demux3/2 -> G4/1
  G4/1 -> Magn-Ang toC3/2
  pickup/1 -> compare1/1
  C to Magn-Ang/1 -> compare1/2, compare/1
  compare1/1 -> Logical Operator/1
  compare/1 -> Logical Operator/2
  Logical Operator/1 -> Out1/1
  Magn-Ang toC/1 -> Sum1/1
  Sum1/1 -> Sum2/1, Sum3/1
  IHA/1 -> Demux/1
  Demux/1 -> Magn-Ang toC/1
  IHB/1 -> Demux1/1
  Demux1/1 -> Magn-Ang toC1/1
  Magn-Ang toC1/1 -> Sum1/2
  IHC/1 -> Demux2/1
  Demux2/1 -> Magn-Ang toC2/1
  Magn-Ang toC2/1 -> Sum1/3
  Demux/2 -> G1/1
  G1/1 -> Magn-Ang toC/2
  Demux1/2 -> G2/1
  G2/1 -> Magn-Ang toC1/2
  Demux2/2 -> G3/1
  G3/1 -> Magn-Ang toC2/2

== system diffrelay/Restricted Earth Relay/Zero Sequence  Overcurrent ==
  In1 : Inport
  Demux3 : Demux  Outputs=2
  Terminator_13 : Terminator
  compare : RelationalOperator  Operator=>  InputSameDT=on
  thro : Constant  Value=zot
  Out1 : Outport
  wires:
  In1/1 -> Demux3/1
  Demux3/2 -> Terminator_13/1
  thro/1 -> compare/2
  compare/1 -> Out1/1
  Demux3/1 -> compare/1

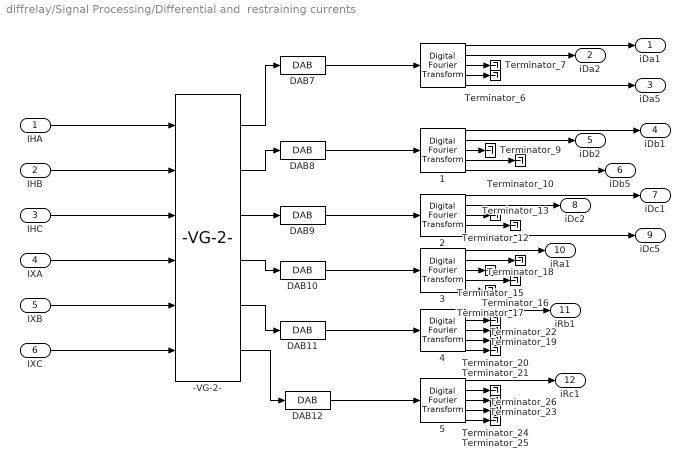
== system diffrelay/Signal Processing/Differential and  restraining currents ==
  IHA : Inport
  IHB : Inport  Port=2
  IHC : Inport  Port=3
  IXA : Inport  Port=4
  IXB : Inport  Port=5
  IXC : Inport  Port=6
   {,1..5} (6 alike) : elements/   fo=60  window_size=32  harmonic=[1 2 3 4 5]
  -VG-2- : elements/-VG-2-  trtype=wye - delta  vector=11  Vh=vp  Vx=vs  nCTH=cth  nCTX=ctx
  DAB{8..12} (5 alike) : elements/DAB  filter=off  approx=Bessel  order=2  numerator=[]  denominator=[]  freq=360  resdis=off  vertres=12  xmax=10  winsize=32  G=1.0  fs=60*32
  DAB7 : elements/DAB  filter=on  approx=Bessel  order=2  numerator=[]  denominator=[]  freq=360  resdis=off  vertres=12  xmax=10  winsize=32  G=1.0  fs=60*32
  Terminator_{6..7,9..10,12..13,15..26} (18 alike) : Terminator
  iDa1 : Outport
  iDa2 : Outport  Port=2
  iDa5 : Outport  Port=3
  iDb1 : Outport  Port=4
  iDb2 : Outport  Port=5
  iDb5 : Outport  Port=6
  iDc1 : Outport  Port=7
  iDc2 : Outport  Port=8
  iDc5 : Outport  Port=9
  iRa1 : Outport  Port=10
  iRb1 : Outport  Port=11
  iRc1 : Outport  Port=12
  wires:
  -VG-2-/1 -> DAB7/1
  -VG-2-/2 -> DAB8/1
  -VG-2-/3 -> DAB9/1
  -VG-2-/4 -> DAB10/1
  -VG-2-/5 -> DAB11/1
  -VG-2-/6 -> DAB12/1
  " 2"/3 -> Terminator_12/1
  " 2"/4 -> Terminator_13/1
  " 4"/5 -> Terminator_21/1
  DAB9/1 -> " 2"/1
  " 5"/2 -> Terminator_26/1
  " 5"/3 -> Terminator_23/1
  " 5"/4 -> Terminator_24/1
  " 5"/5 -> Terminator_25/1
  DAB12/1 -> " 5"/1
  " 4"/3 -> Terminator_19/1
  " 4"/2 -> Terminator_22/1
  DAB11/1 -> " 4"/1
  " 4"/4 -> Terminator_20/1
  " 3"/3 -> Terminator_15/1
  " 3"/4 -> Terminator_16/1
  " 3"/5 -> Terminator_17/1
  " 3"/2 -> Terminator_18/1
  DAB10/1 -> " 3"/1
  " 2"/1 -> iDc1/1
  " 2"/2 -> iDc2/1
  " 2"/5 -> iDc5/1
  " 3"/1 -> iRa1/1
  " 4"/1 -> iRb1/1
  " 5"/1 -> iRc1/1
  IXC/1 -> -VG-2-/6
  IXB/1 -> -VG-2-/5
  IXA/1 -> -VG-2-/4
  IHC/1 -> -VG-2-/3
  IHB/1 -> -VG-2-/2
  IHA/1 -> -VG-2-/1
  " "/4 -> Terminator_6/1
  " "/3 -> Terminator_7/1
  DAB7/1 -> " "/1
  " "/1 -> iDa1/1
  " "/2 -> iDa2/1
  " "/5 -> iDa5/1
  " 1"/3 -> Terminator_9/1
  " 1"/4 -> Terminator_10/1
  " 1"/1 -> iDb1/1
  " 1"/2 -> iDb2/1
  " 1"/5 -> iDb5/1
  DAB8/1 -> " 1"/1

== system diffrelay/Signal Processing/Phasor-magnitude (IR) ==
  IRa1 : Inport
  IRb1 : Inport  Port=2
  IRC1 : Inport  Port=3
  Demux : Demux  Outputs=2
  Demux1 : Demux  Outputs=2
  Demux2 : Demux  Outputs=2
  Terminator_10 : Terminator
  Terminator_8 : Terminator
  Terminator_9 : Terminator
  1 freq. : Outport
  1 freq.1 : Outport  Port=2
  1 freq.2 : Outport  Port=3
  wires:
  Demux/2 -> Terminator_8/1
  Demux/1 -> 1 freq./1
  IRa1/1 -> Demux/1
  Demux1/2 -> Terminator_9/1
  Demux1/1 -> 1 freq.1/1
  IRb1/1 -> Demux1/1
  Demux2/2 -> Terminator_10/1
  Demux2/1 -> 1 freq.2/1
  IRC1/1 -> Demux2/1

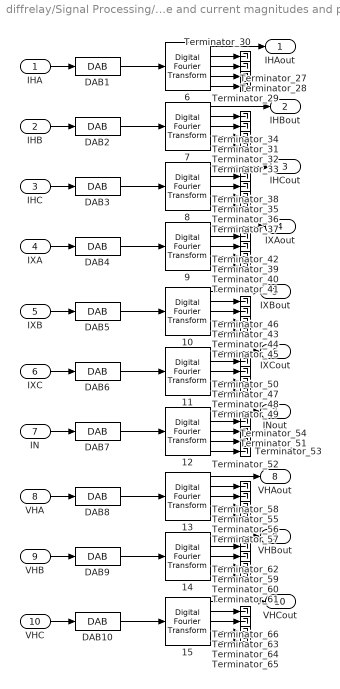
== system diffrelay/Signal Processing/Voltage and current magnitudes and phases ==
  IHA : Inport
  IHB : Inport  Port=2
  IHC : Inport  Port=3
  IXA : Inport  Port=4
  IXB : Inport  Port=5
  IXC : Inport  Port=6
  IN : Inport  Port=7
  VHA : Inport  Port=8
  VHB : Inport  Port=9
  VHC : Inport  Port=10
   {6..15} (10 alike) : elements/   fo=60  window_size=32  harmonic=[1 2 3 4 5]
  DAB{1..10} (10 alike) : elements/DAB  filter=off  approx=Bessel  order=2  numerator=[]  denominator=[]  freq=360  resdis=off  vertres=12  xmax=10  winsize=32  G=1.0  fs=60*32
  Terminator_{27..66} (40 alike) : Terminator
  IHAout : Outport
  IHBout : Outport  Port=2
  IHCout : Outport  Port=3
  IXAout : Outport  Port=4
  IXBout : Outport  Port=5
  IXCout : Outport  Port=6
  INout : Outport  Port=7
  VHAout : Outport  Port=8
  VHBout : Outport  Port=9
  VHCout : Outport  Port=10
  wires:
  " 6"/2 -> Terminator_30/1
  " 6"/3 -> Terminator_27/1
  " 6"/4 -> Terminator_28/1
  " 6"/5 -> Terminator_29/1
  DAB1/1 -> " 6"/1
  IHA/1 -> DAB1/1
  " 7"/2 -> Terminator_34/1
  " 7"/3 -> Terminator_31/1
  " 7"/4 -> Terminator_32/1
  " 7"/5 -> Terminator_33/1
  DAB2/1 -> " 7"/1
  " 8"/2 -> Terminator_38/1
  " 8"/3 -> Terminator_35/1
  " 8"/4 -> Terminator_36/1
  " 8"/5 -> Terminator_37/1
  DAB3/1 -> " 8"/1
  " 9"/2 -> Terminator_42/1
  " 9"/3 -> Terminator_39/1
  " 9"/4 -> Terminator_40/1
  " 9"/5 -> Terminator_41/1
  DAB4/1 -> " 9"/1
  " 10"/2 -> Terminator_46/1
  " 10"/3 -> Terminator_43/1
  " 10"/4 -> Terminator_44/1
  " 10"/5 -> Terminator_45/1
  DAB5/1 -> " 10"/1
  " 11"/2 -> Terminator_50/1
  " 11"/3 -> Terminator_47/1
  " 11"/4 -> Terminator_48/1
  " 11"/5 -> Terminator_49/1
  DAB6/1 -> " 11"/1
  " 12"/2 -> Terminator_54/1
  " 12"/3 -> Terminator_51/1
  " 12"/4 -> Terminator_52/1
  " 12"/5 -> Terminator_53/1
  DAB7/1 -> " 12"/1
  " 13"/2 -> Terminator_58/1
  " 13"/3 -> Terminator_55/1
  " 13"/4 -> Terminator_56/1
  " 13"/5 -> Terminator_57/1
  DAB8/1 -> " 13"/1
  " 14"/2 -> Terminator_62/1
  " 14"/3 -> Terminator_59/1
  " 14"/4 -> Terminator_60/1
  " 14"/5 -> Terminator_61/1
  DAB9/1 -> " 14"/1
  " 15"/2 -> Terminator_66/1
  " 15"/3 -> Terminator_63/1
  " 15"/4 -> Terminator_64/1
  " 15"/5 -> Terminator_65/1
  DAB10/1 -> " 15"/1
  " 6"/1 -> IHAout/1
  " 7"/1 -> IHBout/1
  IHB/1 -> DAB2/1
  " 8"/1 -> IHCout/1
  IHC/1 -> DAB3/1
  " 9"/1 -> IXAout/1
  IXA/1 -> DAB4/1
  " 10"/1 -> IXBout/1
  IXB/1 -> DAB5/1
  " 11"/1 -> IXCout/1
  IXC/1 -> DAB6/1
  " 12"/1 -> INout/1
  IN/1 -> DAB7/1
  " 13"/1 -> VHAout/1
  VHA/1 -> DAB8/1
  " 14"/1 -> VHBout/1
  VHB/1 -> DAB9/1
  " 15"/1 -> VHCout/1
  VHC/1 -> DAB10/1

== system diffrelay/Signal Processing/phasor-magnitude (IDa) ==
  In1 : Inport
  In2 : Inport  Port=2
  In3 : Inport  Port=3
  Demux : Demux  Outputs=2
  Demux1 : Demux  Outputs=2
  Demux2 : Demux  Outputs=2
  Terminator_11 : Terminator
  Terminator_14 : Terminator
  Terminator_8 : Terminator
  1 freq. : Outport
  2 freq. : Outport  Port=2
  5 freq. : Outport  Port=3
  wires:
  In2/1 -> Demux1/1
  In3/1 -> Demux2/1
  In1/1 -> Demux/1
  Demux1/2 -> Terminator_11/1
  Demux2/2 -> Terminator_14/1
  Demux1/1 -> 2 freq./1
  Demux2/1 -> 5 freq./1
  Demux/2 -> Terminator_8/1
  Demux/1 -> 1 freq./1

== system diffrelay/Signal Processing/phasor-magnitude (iDb) ==
  In1 : Inport
  In2 : Inport  Port=2
  In3 : Inport  Port=3
  Demux : Demux  Outputs=2
  Demux1 : Demux  Outputs=2
  Demux2 : Demux  Outputs=2
  Terminator_11 : Terminator
  Terminator_14 : Terminator
  Terminator_8 : Terminator
  1 freq. : Outport
  2 freq. : Outport  Port=2
  5 freq. : Outport  Port=3
  wires:
  Demux1/2 -> Terminator_11/1
  Demux2/2 -> Terminator_14/1
  Demux/2 -> Terminator_8/1
  Demux/1 -> 1 freq./1
  In1/1 -> Demux/1
  Demux1/1 -> 2 freq./1
  In2/1 -> Demux1/1
  Demux2/1 -> 5 freq./1
  In3/1 -> Demux2/1

== system diffrelay/Signal Processing/phasor-magnitude (iDc) ==
  In1 : Inport
  In2 : Inport  Port=2
  In3 : Inport  Port=3
  Demux : Demux  Outputs=2
  Demux1 : Demux  Outputs=2
  Demux2 : Demux  Outputs=2
  Terminator_11 : Terminator
  Terminator_14 : Terminator
  Terminator_8 : Terminator
  1 freq. : Outport
  2 freq. : Outport  Port=2
  5 freq. : Outport  Port=3
  wires:
  In3/1 -> Demux2/1
  Demux2/1 -> 5 freq./1
  In2/1 -> Demux1/1
  Demux1/1 -> 2 freq./1
  In1/1 -> Demux/1
  Demux/1 -> 1 freq./1
  Demux/2 -> Terminator_8/1
  Demux2/2 -> Terminator_14/1
  Demux1/2 -> Terminator_11/1

== system diffrelay/Impedance Relay/ curr1/C to M/A ==
  In1 : Inport
  C to Magn-Ang : ComplexToMagnitudeAngle
  G : Gain  Gain=180/pi  SaturateOnIntegerOverflow=on  OutDataTypeStr=Inherit: Same as input  ParamDataTypeStr=Inherit: Same as input
  Mux1 : Mux  Inputs=2
  Out1 : Outport
  wires:
  C to Magn-Ang/2 -> G/1
  C to Magn-Ang/1 -> Mux1/1
  G/1 -> Mux1/2
  Mux1/1 -> Out1/1
  In1/1 -> C to Magn-Ang/1

== system diffrelay/Impedance Relay/ curr1/C to M/A1 ==
  In1 : Inport
  C to Magn-Ang : ComplexToMagnitudeAngle
  G : Gain  Gain=180/pi  SaturateOnIntegerOverflow=on  OutDataTypeStr=Inherit: Same as input  ParamDataTypeStr=Inherit: Same as input
  Mux1 : Mux  Inputs=2
  Out1 : Outport
  wires:
  In1/1 -> C to Magn-Ang/1
  Mux1/1 -> Out1/1
  G/1 -> Mux1/2
  C to Magn-Ang/1 -> Mux1/1
  C to Magn-Ang/2 -> G/1

== system diffrelay/Impedance Relay/ curr1/C to M/A2 ==
  In1 : Inport
  C to Magn-Ang : ComplexToMagnitudeAngle
  G : Gain  Gain=180/pi  SaturateOnIntegerOverflow=on  OutDataTypeStr=Inherit: Same as input  ParamDataTypeStr=Inherit: Same as input
  Mux1 : Mux  Inputs=2
  Out1 : Outport
  wires:
  C to Magn-Ang/2 -> G/1
  C to Magn-Ang/1 -> Mux1/1
  G/1 -> Mux1/2
  Mux1/1 -> Out1/1
  In1/1 -> C to Magn-Ang/1

== system diffrelay/Impedance Relay/curr2/C to M/A ==
  In1 : Inport
  C to Magn-Ang : ComplexToMagnitudeAngle
  G : Gain  Gain=180/pi  SaturateOnIntegerOverflow=on  OutDataTypeStr=Inherit: Same as input  ParamDataTypeStr=Inherit: Same as input
  Mux1 : Mux  Inputs=2
  Out1 : Outport
  wires:
  C to Magn-Ang/2 -> G/1
  C to Magn-Ang/1 -> Mux1/1
  G/1 -> Mux1/2
  Mux1/1 -> Out1/1
  In1/1 -> C to Magn-Ang/1

== system diffrelay/Impedance Relay/curr2/C to M/A1 ==
  In1 : Inport
  C to Magn-Ang : ComplexToMagnitudeAngle
  G : Gain  Gain=180/pi  SaturateOnIntegerOverflow=on  OutDataTypeStr=Inherit: Same as input  ParamDataTypeStr=Inherit: Same as input
  Mux1 : Mux  Inputs=2
  Out1 : Outport
  wires:
  In1/1 -> C to Magn-Ang/1
  Mux1/1 -> Out1/1
  G/1 -> Mux1/2
  C to Magn-Ang/1 -> Mux1/1
  C to Magn-Ang/2 -> G/1

== system diffrelay/Impedance Relay/curr2/C to M/A2 ==
  In1 : Inport
  C to Magn-Ang : ComplexToMagnitudeAngle
  G : Gain  Gain=180/pi  SaturateOnIntegerOverflow=on  OutDataTypeStr=Inherit: Same as input  ParamDataTypeStr=Inherit: Same as input
  Mux1 : Mux  Inputs=2
  Out1 : Outport
  wires:
  C to Magn-Ang/2 -> G/1
  C to Magn-Ang/1 -> Mux1/1
  G/1 -> Mux1/2
  Mux1/1 -> Out1/1
  In1/1 -> C to Magn-Ang/1

== system diffrelay/Impedance Relay/volt1/C to M/A3 ==
  In1 : Inport
  C to Magn-Ang : ComplexToMagnitudeAngle
  G : Gain  Gain=180/pi  SaturateOnIntegerOverflow=on  OutDataTypeStr=Inherit: Same as input  ParamDataTypeStr=Inherit: Same as input
  Mux1 : Mux  Inputs=2
  Out1 : Outport
  wires:
  In1/1 -> C to Magn-Ang/1
  Mux1/1 -> Out1/1
  G/1 -> Mux1/2
  C to Magn-Ang/1 -> Mux1/1
  C to Magn-Ang/2 -> G/1

== system diffrelay/Impedance Relay/volt1/C to M/A4 ==
  In1 : Inport
  C to Magn-Ang : ComplexToMagnitudeAngle
  G : Gain  Gain=180/pi  SaturateOnIntegerOverflow=on  OutDataTypeStr=Inherit: Same as input  ParamDataTypeStr=Inherit: Same as input
  Mux1 : Mux  Inputs=2
  Out1 : Outport
  wires:
  C to Magn-Ang/2 -> G/1
  C to Magn-Ang/1 -> Mux1/1
  G/1 -> Mux1/2
  Mux1/1 -> Out1/1
  In1/1 -> C to Magn-Ang/1

== system diffrelay/Impedance Relay/volt1/C to M/A5 ==
  In1 : Inport
  C to Magn-Ang : ComplexToMagnitudeAngle
  G : Gain  Gain=180/pi  SaturateOnIntegerOverflow=on  OutDataTypeStr=Inherit: Same as input  ParamDataTypeStr=Inherit: Same as input
  Mux1 : Mux  Inputs=2
  Out1 : Outport
  wires:
  In1/1 -> C to Magn-Ang/1
  Mux1/1 -> Out1/1
  G/1 -> Mux1/2
  C to Magn-Ang/1 -> Mux1/1
  C to Magn-Ang/2 -> G/1

== system diffrelay/Impedance Relay/volt2/C to M/A6 ==
  In1 : Inport
  C to Magn-Ang : ComplexToMagnitudeAngle
  G : Gain  Gain=180/pi  SaturateOnIntegerOverflow=on  OutDataTypeStr=Inherit: Same as input  ParamDataTypeStr=Inherit: Same as input
  Mux1 : Mux  Inputs=2
  Out1 : Outport
  wires:
  C to Magn-Ang/2 -> G/1
  C to Magn-Ang/1 -> Mux1/1
  G/1 -> Mux1/2
  Mux1/1 -> Out1/1
  In1/1 -> C to Magn-Ang/1

== system diffrelay/Impedance Relay/volt2/C to M/A7 ==
  In1 : Inport
  C to Magn-Ang : ComplexToMagnitudeAngle
  G : Gain  Gain=180/pi  SaturateOnIntegerOverflow=on  OutDataTypeStr=Inherit: Same as input  ParamDataTypeStr=Inherit: Same as input
  Mux1 : Mux  Inputs=2
  Out1 : Outport
  wires:
  In1/1 -> C to Magn-Ang/1
  Mux1/1 -> Out1/1
  G/1 -> Mux1/2
  C to Magn-Ang/1 -> Mux1/1
  C to Magn-Ang/2 -> G/1

== system diffrelay/Impedance Relay/volt2/C to M/A8 ==
  In1 : Inport
  C to Magn-Ang : ComplexToMagnitudeAngle
  G : Gain  Gain=180/pi  SaturateOnIntegerOverflow=on  OutDataTypeStr=Inherit: Same as input  ParamDataTypeStr=Inherit: Same as input
  Mux1 : Mux  Inputs=2
  Out1 : Outport
  wires:
  C to Magn-Ang/2 -> G/1
  C to Magn-Ang/1 -> Mux1/1
  G/1 -> Mux1/2
  Mux1/1 -> Out1/1
  In1/1 -> C to Magn-Ang/1
